simulink model "fc_alone_with_temp"  (R2020b)
settings: Solver=VariableStepAuto  StartTime=0.0  StopTime=10.0  RelTol=1e-3
undefined symbols (not defined in the file or in its folder): DiscIntNeverNeededParam, Ts
libraries: powerlib x6, simulink x2
settings Model: Creator=maloc  LastModifiedBy=maloc

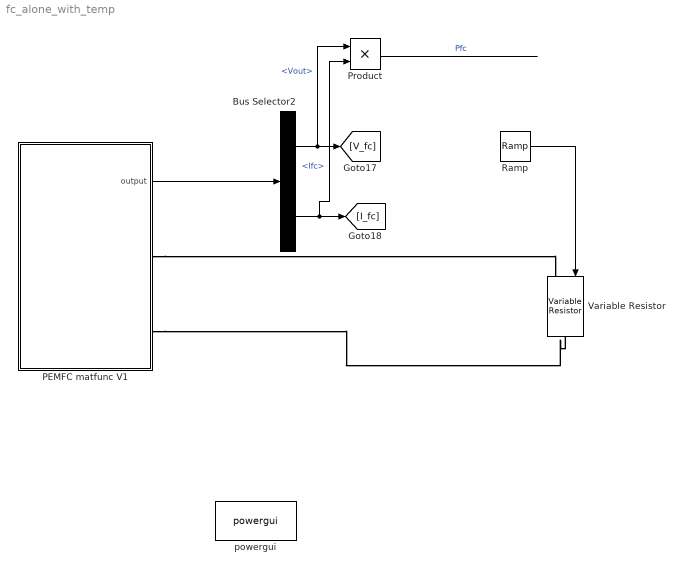
== system fc_alone_with_temp ==
  Bus Selector2 : BusSelector  OutputSignals=Vout,Ifc
  PEMFC matfunc V1 : Subsystem  mask{P_H2=0.5, P_O2=1, T=313.15, W=14, tm=1.27e-4, Nfc=50, Rohm=0.061871, Ts=Ts, fc_tau=1}
      mask prompts: P_H2 "Hydrogen pressure (atm)"; P_O2 "Oxygen pressure (atm)"; T "Temperature (K)"; W "Water Content"; tm "Thickness of the membrane (m)"; Nfc "Number of cells"; Rohm "Fuel cell resistance"; Ts "Sample time (s)"; fc_tau "Dynamic response of the FC (s)"
      mask init:
      | tau = fc_tau / 5;
  Product : Product
  Ramp : simulink/Sources/Ramp  slope=1  start=0  InitialOutput=1
  Variable Resistor : powerlib/Elements/Variable Resistor  Rabsmin=1e-3
      settings: SourceProductBaseCode=PS
  powergui : powerlib/powergui  Priority=1  SimulationMode=Discrete  SampleTime=1e-3  frequency=60  Iterations=50  frequencyindice=0  Pbase=100e6  ErrMax=1e-4  UnitsV=kV  UnitsW=MW  buscounter=0  FunctionMessages=off  echomessages=off  EnableUseOfTLC=off  CurrentSourceSwitches=off  DisableSnubberDevices=off  DisableRonSwitches=off  DisableVfSwitches=off  DisplayEquations=off  AutomaticDiscreteSolvers=off  SolverType=Tustin/Backward Euler (TBE)  Interpol=off  ExternalGateDelay=off  methode=off  Ts=100  x0status=blocks  SPID=on  SwTol=0  HookPort=off  NonlinearTolerance=1e-4  nMaxIteration=100  ContinueOnMaxIteration=off  RestoreLinks=warning  ResistiveCurrentMeasurement=off  Frange=[0:2:500]  Ylog=off  Xlog=on  ShowGrid=off  save=off  variable=ZData  structure=0  ZoomFFT=off  StartTime=0.0  cycles=1  DisplayStyle=1  fundamental=60  FreqAxis=off  MaxFrequency=1000  frequencyindicesteady=1  RmsSteady=1  display=off
  wires:
  Bus Selector2/1 -> Product/1, [V_fc]  "<Vout>"
  PEMFC matfunc V1/1(output) -> Bus Selector2/1
  Bus Selector2/2 -> Product/2, [I_fc]  "<Ifc>"
  Ramp/1 -> Variable Resistor/1
  Product/1 -> ?  "Pfc"
  connections:
  PEMFC matfunc V1/RConn2 -- Variable Resistor/RConn1
  PEMFC matfunc V1/RConn1 -- Variable Resistor/LConn1

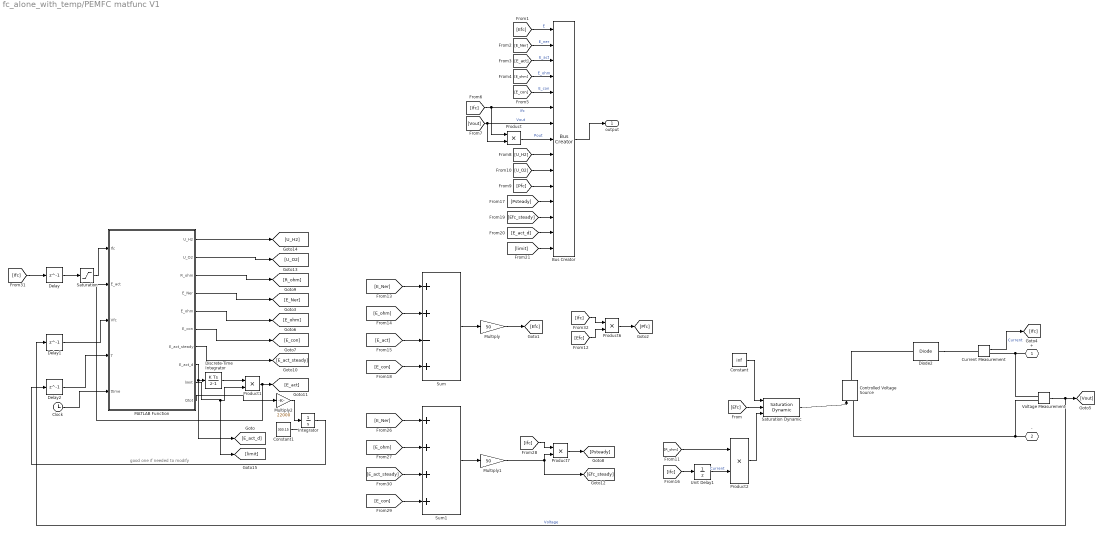
== system fc_alone_with_temp/PEMFC matfunc V1 ==
  note: good one if needed to modify
  Bus Creator : BusCreator  Inputs=15
  Clock : Clock
  Constant : Constant  Value=inf
  Constant1 : Constant  Value=303.15
  Controlled Voltage Source : powerlib/Electrical Sources/Controlled Voltage Source  Initialize=on  Source_Type=AC  Amplitude=0  Phase=0  Frequency=0  Measurements=None
  Current Measurement : powerlib/Measurements/Current Measurement  PhasorSimulation=off  OutputType=Complex  PSBequivalent=0
  Delay : Delay  DelayLength=1
  Delay1 : Delay  DelayLength=1
  Delay2 : Delay  DelayLength=1
  Diode2 : powerlib/Power Electronics/Diode  Ron=Rohm  Lon=0  Vf=0  IC=0  UseSnubber=off  Rs=1e4  Cs=inf  Measurements=off
  Discrete-Time Integrator : DiscreteIntegrator  SampleTime=-1  ICPrevOutput=DiscIntNeverNeededParam  ICPrevScaledInput=DiscIntNeverNeededParam
  Integrator : Integrator
  MATLAB Function : MATLAB Function  TreatAsAtomicUnit=on
  Multiply : Gain  Gain=50
  Multiply1 : Gain  Gain=50
  Multiply2 : Gain  Gain=22000
  Product{,1..2,6..7} (5 alike) : Product
  Saturation : Saturate  UpperLimit=inf  LowerLimit=0.001
  Saturation Dynamic : simulink/Discontinuities/Saturation Dynamic  OutMin=[]  OutMax=[]  OutDataTypeStr=Inherit: Same as second input  OutDataType=fixdt(1, 16)  OutScaling=2^-10  DoSatur=off
  Sum : Sum  Inputs=++-+
  Sum1 : Sum  Inputs=++++
  Unit Delay1 : UnitDelay  SampleTime=Ts  HasFrameUpgradeWarning=on
  Voltage Measurement : powerlib/Measurements/Voltage Measurement  PhasorSimulation=off  OutputType=Complex  PSBequivalent=0
  + : PMIOPort  Tag=PMCPort  Side=Right
  - : PMIOPort  Tag=PMCPort  Port=2  Side=Right
  output : Outport  VectorParamsAs1DForOutWhenUnconnected=off
  wires:
  [Efc] -> Bus Creator/1  "E"
  [E_Ner] -> Bus Creator/2  "E_ner"
  [E_act] -> Bus Creator/3  "E_act"
  [E_ohm] -> Bus Creator/4  "E_ohm"
  [Ifc] -> Product/1, Bus Creator/6  "Ifc"
  [Vout] -> Product/2, Bus Creator/7  "Vout"
  [E_con] -> Bus Creator/5  "E_con"
  Product/1 -> Bus Creator/8  "Pout"
  Current Measurement/1 -> [Ifc]  "Current"
  Voltage Measurement/1 -> Delay1/1, [Vout]  "Voltage"
  [U_H2] -> Bus Creator/9
  [U_O2] -> Bus Creator/10
  Bus Creator/1 -> output/1
  [Ifc] -> Unit Delay1/1
  Unit Delay1/1 -> Product2/2  "Current"
  Product2/1 -> Saturation Dynamic/3
  [R_ohm] -> Product2/1
  Constant/1 -> Saturation Dynamic/1
  Saturation Dynamic/1 -> Controlled Voltage Source/1
  MATLAB Function/3(R_ohm) -> [R_ohm]
  MATLAB Function/7(E_act_steady) -> [E_act_steady]
  MATLAB Function/5(E_ohm) -> [E_ohm]
  Discrete-Time Integrator/1 -> Product1/1
  [Efc] -> Product6/2
  [E_ohm] -> Sum1/2
  Multiply1/1 -> [Efc_steady], Product7/2
  [E_con] -> Sum1/4
  [Ifc] -> Product7/1
  [E_ohm] -> Sum/2
  [E_act] -> Sum/3
  Product6/1 -> [Pfc]
  [E_act_steady] -> Sum1/3
  Sum1/1 -> Multiply1/1
  Sum/1 -> Multiply/1
  MATLAB Function/4(E_Ner) -> [E_Ner]
  [E_con] -> Sum/4
  MATLAB Function/6(E_con) -> [E_con]
  [Ifc] -> Product6/1
  [E_Ner] -> Sum1/1
  [Ifc] -> Delay/1
  Multiply/1 -> [Efc]
  MATLAB Function/8(E_act_d) -> [E_act_d], Discrete-Time Integrator/1
  [E_Ner] -> Sum/1
  [Efc] -> Saturation Dynamic/2
  Product7/1 -> [Psteady]
  [Efc_steady] -> Bus Creator/13
  [Pfc] -> Bus Creator/11
  [Psteady] -> Bus Creator/12
  MATLAB Function/1(U_H2) -> [U_H2]
  MATLAB Function/2(U_O2) -> [U_O2]
  Saturation/1 -> MATLAB Function/1(Ifc)
  Delay/1 -> Saturation/1
  Product1/1 -> MATLAB Function/2(E_act), [E_act]
  MATLAB Function/9(limit) -> [limit], Product1/2
  [E_act_d] -> Bus Creator/14
  [limit] -> Bus Creator/15
  Constant1/1 -> ?
  MATLAB Function/10(Qtot) -> Multiply2/1
  Delay1/1 -> MATLAB Function/3(Vfc)
  Delay2/1 -> MATLAB Function/4(T)
  Integrator/1 -> Delay2/1
  Multiply2/1 -> Integrator/1
  Clock/1 -> MATLAB Function/5(ttime)
  connections:
  -/RConn1 -- Voltage Measurement/LConn2 -- Controlled Voltage Source/LConn1
  +/RConn1 -- Voltage Measurement/LConn1 -- Current Measurement/RConn1
  Diode2/RConn1 -- Current Measurement/LConn1
  Diode2/LConn1 -- Controlled Voltage Source/RConn1

== matlab function fc_alone_with_temp/PEMFC matfunc V1/MATLAB Function ==
  settings: updateMethod=DISCRETE  sampleTime=Ts
  data: U_H2 output; U_O2 output; R_ohm output; Ifc input; E_Ner output; E_ohm output; E_con output; E_act_steady output; E_act input; E_act_d output; limit output; Vfc input; T input; Qtot output; ttime input
function [U_H2,U_O2,R_ohm,E_Ner,E_ohm,E_con,E_act_steady,E_act_d,limit,Qtot] = fcn(Ifc,E_act,Vfc,T,ttime)
%     https://link.springer.com/article/10.1007/s40565-016-0196-5
%     Modeling and Simulation of a Proton Exchange Membrane Fuel Cell Alongside a Waste Heat Recovery System Based on the Organic Rankine Cycle in MATLAB/SIMULINK Environment
%     MATHEMATICAL MODELLING FOR PROTON EXCHANGE MEMBRANE FUEL CELL (PEMFC) 
%     https://www.scirp.org/pdf/epe_2020112310053180.pdf#page=17&zoom=100,72,604
%     H-Series Fuel Cell Stacks
% https://ieeexplore.ieee.org/document/6243436
% https://www.scirp.org/journal/paperinformation.aspx?paperid=84317




    %% constants:
    Tamb = 303.15; 
    R = 8.3145;
    Pstd = 101325;
    nF = 2*96485;
    C_act = 2;
    A = 19.6*4.0;
%     T = 303.15;
    Nfc = 50;
    lambda = 14;
    l = 21e-4 * 10^-2;
%     l = 1.27e-4;
    CpH2 = 28.68;
    CpO2 = 29.39;
    CpH2O = 75.4;
    HvH2O = 40644;
    
    
% if T == 0
%     T = 303.15;
% else
%     T = T + 303.15;
% end
% T
% qcell = -Nfc*Ifc*1.229;
% qelec = Vfc*Ifc;
% qsens = (T-Tamb)*((Ifc/nF*CpH2)+(Ifc/2/nF*CpO2)+(Ifc/nF*CpH2O))+(Ifc/nF*HvH2O);
% % qconv = 37.5*(T-Tamb)*Nfc*A*1e-6;
% qconv = 0;
% Qtot = qcell - qelec - qsens - qconv;
% [qcell, qsens, qconv, Qtot]
Qtot = 0;
    Tamb = 303.15;
    if ttime > 5
        Tamb = 273;
    end
    p1 = -0.03802;
    p2 = 0.5095;
    p3 = 172.6;
    p4 = 1.1;
    p5 = 27.56;
    tau = p1*Ifc^2+p2*Ifc+p3;
    T = Tamb + ((p4*Ifc + p5)-Tamb)*(1-exp(-ttime/tau));

    J = Ifc/A;
    JM = 45/A;
    Pa = 1.45;
    Pc = 1;
    Tc = T-273.15;
    coeff = 1.05;
        
%     if Ifc <=0
%         Ifc = 40;
%     end
    
    PH2Osat = 10^(-2.18+2.95e-2*Tc-9.18e-5*Tc^2+1.44e-7*Tc^3);
    
    P_H2 = 0.5*PH2Osat*(exp(-(1.635*J/T^1.334))*(Pa/PH2Osat)-1);
    P_O2 = PH2Osat*(exp(-(4.192*J/T^1.334))*(Pc/PH2Osat)-1);
    

    %% Saturation at start
    if -1.87e-4*log(Ifc) > 0
        k = 0;
    else
        if -1.87e-4*log(Ifc) < -1.2
            k = -1.2;
        else
            k = -1.87e-4*log(Ifc);
        end
    end
    %% Nernst Voltage
    E_Ner = 1.229 + (T-298.15) * (-0.85e-3) + T*R/nF * log(P_H2*P_O2^0.5);
    
    %% Activation loss
    % Pressure not in Pa ?
    CO2 = (P_O2/(5.08e6))*exp(498/T);
%     CH2 = (P_H2/(1.09e6))*exp(-77/T);
%     E_act_steady=-0.9514 + T * (2.86e-3+2.1e-4*log(200)+4.3e-5*log(CH2)+7.4e-5*log(CO2)+k);
    E_act_steady = -0.9514 + 3.12e-3*T + 7.4e-5*T*log(CO2) -1.87e-4*T*log(Ifc);
    
    %% Ohmic loss
%     E_ohm = - Ifc*(l/((lambda*5.139e-3-3.26e-3)*exp(1268*(1/303-1/T))));
    R_ohm = (l/((lambda*5.139e-3-3.26e-3)*exp(1268*(1/303-1/T))));
    E_ohm = -Ifc*l/A*(181.6*(1+0.03*(Ifc/A))+0.062*(T/303)^2*(Ifc/A)^2.5)/((lambda-0.634-3*(Ifc/A))*exp(4.18*((T-303)/T)));
    
    %% Concentration loss
%     if T>= 312.15
%         E_con = (1.1e-4-1.2e-6*(T-273.15))*exp(8*Ifc/40);
%     else
%         E_con = (3.3e-3-8.2e-5*(T-273.15))*exp(8*Ifc/40);
%     end

%     E_con = 3*R*T/(2*nF)*log(1-J/JM)-1.5607*R*T/(2*nF);
    if J/JM < 1
        E_con = 3*R*T/(2*nF)*log(1-J/JM)-1.5607*R*T/(2*nF);
    else
%         E_con = -abs(3*R*T/(2*nF)*log(complex(1-J/(JM-0.001)))-1.5607*R*T/(2*nF));
        E_con = 3*R*T/(2*nF)*log(J/JM)-1.5607*R*T/(2*nF);
    end
    
    %% with coefficient
    E_con = coeff * E_con;
    E_act_steady = coeff * E_act_steady;
    E_ohm = coeff * E_ohm;
    E_Ner = coeff * E_Ner;
    
        
    %% activation dynamic loss:
    below = -E_act_steady-E_con;
    E_act_d = (Ifc/C_act)*(1-E_act/below);
%     E_act_d = 0;

    %% Fuel utilization
    U_H2 = 60000*Ifc*R*T*Nfc/(nF*1.16*1*0.9995*Pstd);
    
    %% Air utilization
    U_O2 = 60000*Ifc*R*T*Nfc/(2*nF*0.0181*1*0.21*Pstd);
    limit = 1;
%     if J/JM >= 1
%             E_con = 0;
%             E_act_steady = 0;
%             E_ohm = 0;
%             E_act_d = 0;
%             E_Ner = -35*Ifc;
%             if E_Ner <= 0
%                 E_Ner = 0;
%             end
%             limit = 0;
%     end
    
    
    %%
    
    
end
